simulink library "library"  (R2017a)
settings: Solver=VariableStepAuto  StartTime=0.0  StopTime=10.0  RelTol=1e-3
settings Model: Creator=ibrahim  LastModifiedBy=ibrahim

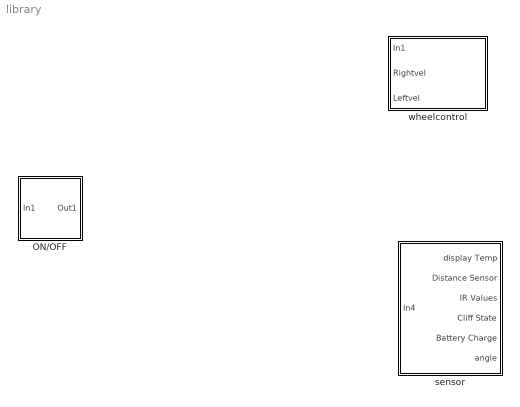
== system library ==
  ON/OFF : Subsystem
  sensor : Subsystem  TreatAsAtomicUnit=on
      settings: PermitHierarchicalResolution=None
  wheelcontrol : Subsystem  AncestorBlock=mylibrary/wheelcontrol

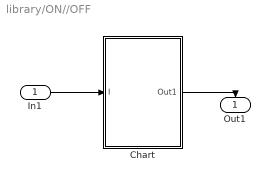
== system library/ON//OFF ==
  In1 : Inport
  Chart : Stateflow chart  TreatAsAtomicUnit=on
  Out1 : Outport
  wires:
  Chart/1(Out1) -> Out1/1
  In1/1 -> Chart/1(I)

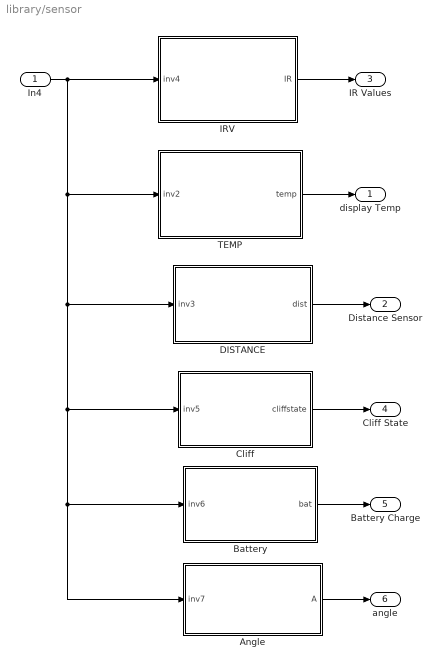
== system library/sensor ==
  In4 : Inport
  Angle : Stateflow chart  TreatAsAtomicUnit=on
  Battery : Stateflow chart  TreatAsAtomicUnit=on
  Cliff : Stateflow chart  TreatAsAtomicUnit=on
  DISTANCE : Stateflow chart  TreatAsAtomicUnit=on
  IRV : Stateflow chart  TreatAsAtomicUnit=on
  TEMP : Stateflow chart  TreatAsAtomicUnit=on
  display Temp : Outport
  Distance Sensor : Outport  Port=2
  IR Values : Outport  Port=3
  Cliff State : Outport  Port=4
  Battery Charge : Outport  Port=5
  angle : Outport  Port=6
  wires:
  TEMP/1(temp) -> display Temp/1
  IRV/1(IR) -> IR Values/1
  DISTANCE/1(dist) -> Distance Sensor/1
  In4/1 -> Angle/1(inv7), Battery/1(inv6), Cliff/1(inv5), DISTANCE/1(inv3), TEMP/1(inv2), IRV/1(inv4)
  Cliff/1(cliffstate) -> Cliff State/1
  Angle/1(A) -> angle/1
  Battery/1(bat) -> Battery Charge/1

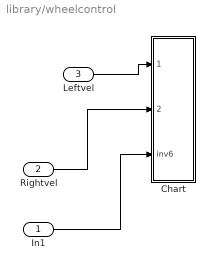
== system library/wheelcontrol ==
  In1 : Inport
  Rightvel : Inport  Port=2
  Leftvel : Inport  Port=3
  Chart : Stateflow chart  TreatAsAtomicUnit=on
  wires:
  Leftvel/1 -> Chart/1(Leftvel)
  Rightvel/1 -> Chart/2(Rightvel)
  In1/1 -> Chart/3(inv6)

== stateflow chart library/ON//OFF/Chart ==
  state init
    en:
    tcpinit;
    Out1=1;
  state TurnRoombaOff
    en:
    OFF;
    Out1=0;
  (default) -> init
  TurnRoombaOff -> init : [I==1]
  init -> TurnRoombaOff : [I==0]
  data: Out1 output; I input
  function tcpinit:
    | function tcpinit
    | coder.extrinsic('RoombaInit_wifi');
    | coder.extrinsic('assignin');
    | persistent tcpobj
    | tcpobj=RoombaInit_wifi('10.0.0.1','full');
    | assignin('base','ha',tcpobj);
  function OFF:
    | function OFF
    | persistent sl
    | 
    | coder.extrinsic('evalin');
    | coder.extrinsic('get');
    | sl = evalin('base','ha');
    | coder.extrinsic('PowerOffRoomba')
    | PowerOffRoomba(sl);

== stateflow chart library/sensor/Cliff ==
  state on
    en,du:
    cliffstate=CliffState;
  state off
    en,du:
    cliffstate=[0,0,0,0];
  (default) -> off
  on -> off : [inv5==0]
  off -> on : [inv5==1]
  data: y function_output; cliffstate output; inv5 input
  function y=CliffState:
    | function y=CliffState
    | persistent so4
    | y=zeros(1,4);
    | coder.extrinsic('evalin');
    | coder.extrinsic('get');
    | so4 = evalin('base','ha');
    | csr=[0,0,0,0];
    | coder.extrinsic('CliffStateRoomba');
    | csr= CliffStateRoomba(so4);
    | y=csr;

== stateflow chart library/sensor/Battery ==
  state on
    en,du:
    bat=battery;
  state off
    en,du:
    bat=0;
  (default) -> off
  off -> on : [inv6==1]
  on -> off : [inv6==0]
  data: y function_output; inv6 input; bat output
  function y=battery:
    | function y=battery
    | persistent so5
    | y=0;
    | coder.extrinsic('evalin');
    | coder.extrinsic('get');
    | so5 = evalin('base','ha');
    | B=0;
    | coder.extrinsic('BatteryChargeReaderRoomba_me');
    | B= BatteryChargeReaderRoomba_me(so5);
    | y=B;

== stateflow chart library/sensor/Angle ==
  state on
    en,du:
    A=Angle;
  state off
    en,du:
    A=0;
  (default) -> off
  off -> on : [inv7==1]
  on -> off : [inv7==0]
  data: y function_output; inv7 input; A output
  function y=Angle:
    | function y=Angle
    | persistent so6
    | y=0;
    | A=0;
    | coder.extrinsic('AngleSensorRoomba');
    | coder.extrinsic('evalin');
    | coder.extrinsic('get');
    | so6 = evalin('base','ha');
    | A= AngleSensorRoomba(so6);
    | 
    | y=A;

== stateflow chart library/sensor/IRV ==
  state on
    en,du:
    IR=IRV;
  state off
    en,du:
    IR=zeros(1,6);
  (default) -> off
  off -> on : [inv4==1]
  on -> off : [inv4==0]
  data: y function_output; IR output; inv4 input
  function y= IRV:
    | function y= IRV
    | persistent so1
    | y=zeros(1,6);
    | coder.extrinsic('evalin');
    | 
    |     so1 = evalin('base','ha');
    | 
    | IR = zeros(1, 6);
    | coder.extrinsic('RangeStateRoomba');
    | IR = RangeStateRoomba(so1);
    | y=IR;

== stateflow chart library/sensor/TEMP ==
  state off
    en,du:
    temp=0;
  state on
    en,du:
    temp=T;
  (default) -> off
  off -> on : [inv2==1]
  on -> off : [inv2==0]
  data: y function_output; inv2 input; temp output
  function y= T:
    | function y= T
    | persistent so2
    | y=1;
    | coder.extrinsic('evalin');
    | coder.extrinsic('get');
    | so2 = evalin('base','ha');
    | temp=0;  
    | coder.extrinsic('TemperatureRoomba');
    | temp=TemperatureRoomba(so2);
    | 
    | y=temp;

== stateflow chart library/sensor/DISTANCE ==
  state on
    en,du:
    dist=Distance;
  state off
    en,du:
    dist=0;
  (default) -> off
  off -> on : [inv3==1]
  on -> off : [inv3==0]
  data: y function_output; inv3 input; dist output
  function y=Distance:
    | function y=Distance
    | persistent so3
    | y=0;
    | coder.extrinsic('evalin');
    | coder.extrinsic('get');
    | so3 = evalin('base','ha');
    | dist=0;
    | coder.extrinsic('DistanceSensorRoomba');
    | dist= DistanceSensorRoomba(so3);
    | y=dist;

== stateflow chart library/wheelcontrol/Chart ==
  state wheel
    en,du:
    tcpget3(Rightvel,Leftvel);
  state off
    en,du:
  (default) -> off
  wheel -> off : [inv6==0]
  off -> wheel : [inv6==1]
  data: u1 function_input; u2 function_input; Leftvel input; Rightvel input; inv6 input
  function tcpget3(u1,u2):
    | function tcpget3(u1,u2)
    | persistent so
    | coder.extrinsic('evalin');
    | coder.extrinsic('get');
    | so = evalin('base','ha');
    | coder.extrinsic('SetWheelVelRoomba');
    | SetWheelVelRoomba(so,u1 , u2);
